simulink model "NN_2"  (R2024a)
settings: Solver=VariableStepAuto  StartTime=0.0  StopTime=7  RelTol=1e-3
libraries: roblocks x3
settings Model: Creator=nicolasaltarelli  LastModifiedBy=nicolasaltarelli
settings DataIOCC: ReturnWorkspaceOutputs=off
settings RTWCC: GPUComputeCapability=3.5

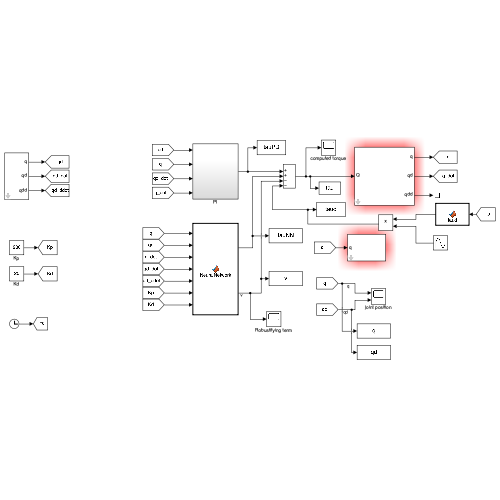
[thumbnail: Simulink's stored preview of the top-level diagram]
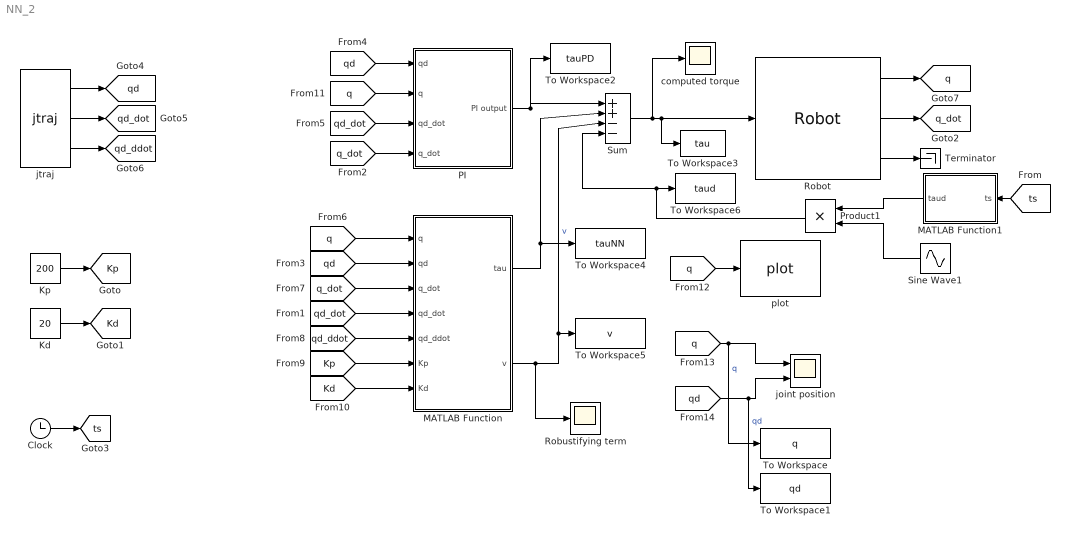
== system NN_2 ==
  Clock : Clock
  Kd : Constant  Value=20
  Kp : Constant  Value=200
  MATLAB Function : MATLAB Function  TreatAsAtomicUnit=on
  MATLAB Function1 : MATLAB Function  TreatAsAtomicUnit=on
  PI : Subsystem
  Product1 : Product
  Robot : roblocks/Arm/Robot  robot=p560.nofriction  q0=[0 0 0 0 0 0]
  Robustifying term : Scope
  Sine Wave1 : Sin  SampleTime=0
  Sum : Sum  Inputs=|++--
  Terminator : Terminator
  To Workspace : ToWorkspace  VariableName=q  SaveFormat=Timeseries  SampleTime=-1
  To Workspace1 : ToWorkspace  VariableName=qd  SaveFormat=Timeseries  SampleTime=-1
  To Workspace2 : ToWorkspace  VariableName=tauPD  SaveFormat=Timeseries  SampleTime=-1
  To Workspace3 : ToWorkspace  VariableName=tau  SaveFormat=Timeseries  SampleTime=-1
  To Workspace4 : ToWorkspace  VariableName=tauNN  SaveFormat=Timeseries  SampleTime=-1
  To Workspace5 : ToWorkspace  VariableName=v  SaveFormat=Timeseries  SampleTime=-1
  To Workspace6 : ToWorkspace  VariableName=taud  SaveFormat=Timeseries  SampleTime=-1
  computed torque : Scope
  joint position : Scope  NumInputPorts=2
  jtraj : roblocks/Toolbox/jtraj  q0=[0 0 0 0 0 0]  qf=[-pi/6 -pi/3 -pi/2 0 0 0]  tmax=5  ts=-1
  plot : roblocks/Arm/plot  robot=p560  fps=25  holdplot=on
  tag scope: Kd=global, Kp=global, q=global, q_dot=global, qd=global, qd_ddot=global, qd_dot=global, ts=global
  wires:
  Robot/3 -> Terminator/1
  Sum/1 -> computed torque/1, To Workspace3/1, Robot/1
  Robot/1 -> [q]
  Robot/2 -> [q_dot]
  [qd] -> PI/1(qd)
  [q] -> PI/2(q)
  [qd_dot] -> PI/3(qd_dot)
  [q_dot] -> PI/4(q_dot)
  PI/1(PI output) -> To Workspace2/1, Sum/1
  [q] -> MATLAB Function/1(q)
  [qd] -> MATLAB Function/2(qd)
  [q_dot] -> MATLAB Function/3(q_dot)
  [qd_dot] -> MATLAB Function/4(qd_dot)
  [qd_ddot] -> MATLAB Function/5(qd_ddot)
  [Kp] -> MATLAB Function/6(Kp)
  [Kd] -> MATLAB Function/7(Kd)
  [q] -> plot/1
  [q] -> To Workspace/1, joint position/1  "q"
  [qd] -> To Workspace1/1, joint position/2  "qd"
  MATLAB Function/2(v) -> Sum/3, To Workspace5/1, Robustifying term/1  "v"
  Kp/1 -> [Kp]
  jtraj/2 -> [qd_dot]
  jtraj/1 -> [qd]
  jtraj/3 -> [qd_ddot]
  Kd/1 -> [Kd]
  MATLAB Function/1(tau) -> To Workspace4/1, Sum/2
  Product1/1 -> Sum/4, To Workspace6/1
  MATLAB Function1/1(taud) -> Product1/1
  Sine Wave1/1 -> Product1/2
  Clock/1 -> [ts]
  [ts] -> MATLAB Function1/1(ts)

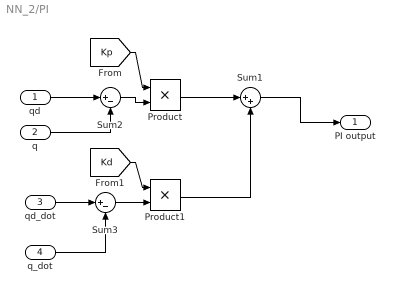
== system NN_2/PI ==
  qd : Inport
  q : Inport  Port=2
  qd_dot : Inport  Port=3
  q_dot : Inport  Port=4
  Product : Product
  Product1 : Product
  Sum1 : Sum  Inputs=|++
  Sum2 : Sum  Inputs=|+-
  Sum3 : Sum  Inputs=|+-
  PI output : Outport
  wires:
  Sum1/1 -> PI output/1
  qd_dot/1 -> Sum3/1
  q/1 -> Sum2/2
  Sum2/1 -> Product/2
  qd/1 -> Sum2/1
  q_dot/1 -> Sum3/2
  Sum3/1 -> Product1/2
  Product/1 -> Sum1/1
  [Kp] -> Product/1
  Product1/1 -> Sum1/2
  [Kd] -> Product1/1

== matlab function NN_2/MATLAB Function1 ==
  data: ts input; taud output
function taud = taud(ts)
if ts>=2 && ts<=5
    taud = 5*[-0.1384 -0.8396 1.3546 0 0 0]';
else
    taud = [0 0 0 0 0 0]';
end

== matlab function NN_2/MATLAB Function ==
  settings: updateMethod=DISCRETE
  data: q input; tau output; qd input; q_dot input; qd_dot input; qd_ddot input; Kp input; Kd input; v output
function [tau,v] = NeuralNetwork(q, qd, q_dot, qd_dot, qd_ddot,Kp,Kd)
    e = qd - q;
    e_dot = qd_dot - q_dot;
    Lambda = Kp/Kd * eye(6);
    r = Lambda*e + e_dot; 
    
    x = [1; e; e_dot; qd; qd_dot; qd_ddot];
    state_dim = length(q);
    hidden_dim = 5 * state_dim;

    ki = 0.10;

    persistent W V
    if isempty(W) || isempty(V)
        W = randn(hidden_dim+1, state_dim) * 0.1;
        V = randn(length(x), hidden_dim) * 0.1;
    end

    F = 0.1;
    G = 0.4;
    
    activation = @(x) tanh(x);
    activation_derivative = @(x) 1 - tanh(x).^2;
    
    sigma = activation(V' * x);
    f_hat = W' * [1;sigma];
    
    tau = f_hat;
    
    sigma_prime = diag(activation_derivative(V' * x));    
    V = V + G * (x * (sigma_prime * (W(2:end, :) * r))') -ki*G*norm(r)*V;
    W = W + F * ([1;sigma] * r') - F*[zeros(1, state_dim); sigma_prime * (V'*x*r')] - ki*F*norm(r)*W ; 
    
    Z = [W zeros(hidden_dim+1,hidden_dim); zeros(length(x),state_dim) V];

    norm_Zf = norm(Z, 'fro'); 
    Z_b = 1.1*norm_Zf;
    C2 = 0.07*Z_b;
    Kz = 1.2*C2;
    
    v = -Kz*(norm_Zf + Z_b)*r;

end
